simulink model "raspberrypi_I2C_temp_init"  (R2018b)
settings: Solver=FixedStepAuto  StartTime=0.0  StopTime=inf  RelTol=1e-3
undefined symbols (not defined in the file or in its folder): Green, led0
libraries: raspberrypilib x3, embdlinuxlib x1, realtime_examples_misc x1
settings Model: SimulationMode=external  ExtModeTrigDuration=2  Creator=The MathWorks, Inc.  LastModifiedBy=The MathWorks, Inc.
settings SolverCC: PositivePriorityOrder=on
settings DataIOCC: LimitDataPoints=on
settings OptimizationCC: BlockReduction=off  LifeSpan=Inf  MaxStackSize=64
settings DebuggingCC: AllowSymbolicDim=off  SFUnexpectedBacktrackingDiag=warning  SFNoUnconditionalDefaultTransitionDiag=warning  SFExecutionAtInitializationDiag=none
settings HardwareCC: ProdBitPerPointer=32  ProdBitPerSizeT=32  ProdBitPerPtrDiffT=32  ProdLargestAtomicInteger=Long  ProdLargestAtomicFloat=Double  ProdWordSize=32  ProdHWDeviceType=ARM Compatible->ARM Cortex  UseEmbeddedCoderFeatures=off  UseSimulinkCoderFeatures=off
settings ModelReferenceCC: PropagateSignalLabelsOutOfModel=off
settings SFSimCC: SimUseLocalCustomCode=off
settings RTWCC: SystemTargetFile=ert.tlc  HardwareBoard=Raspberry Pi  TemplateMakefile=ert_default_tmf  RTWUseLocalCustomCode=off  Toolchain=GNU GCC Raspberry Pi  BuildConfiguration=Faster Runs
settings CodeAppCC: StateflowObjectComments=on
settings ERTTargetCC: MultiwordLength=2048  ERTCustomFileBanners=off  SupportContinuousTime=on  SupportNonInlinedSFcns=on  RemoveResetFunc=off  SupportVariableSizeSignals=on  ModelStepFunctionPrototypeControlCompliant=off  ConvertIfToSwitch=off  SuppressUnreachableDefaultCases=off
settings ConfigComp: CovMetricSettings=dw  CovHtmlReporting=on  CovSaveCumulativeToWorkspaceVar=on  CovSaveSingleToWorkspaceVar=on  CovExternalEMLEnable=off

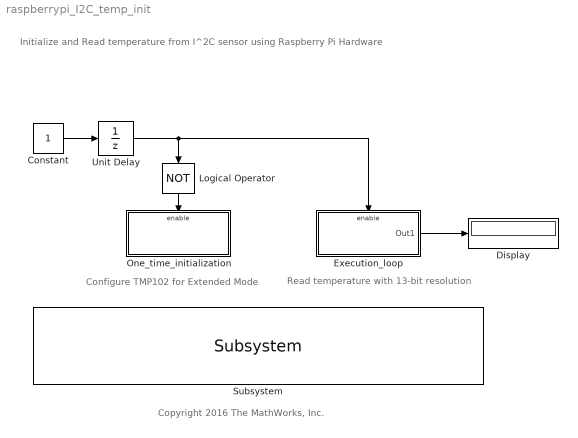
== system raspberrypi_I2C_temp_init ==
  note: Read temperature with 13-bit resolution
  note: Configure TMP102 for Extended Mode
  note: Copyright 2016 The MathWorks, Inc.
  note: Initialize and Read temperature from I^2C sensor
      |  using Raspberry Pi Hardware
  Constant : Constant  OutDataTypeStr=boolean  SampleTime=0.1
  Display : Display
  Execution_loop : Subsystem  TreatAsAtomicUnit=on
  Logical Operator : Logic  Operator=NOT  AllPortsSameDT=off  OutDataTypeStr=boolean
  One_time_initialization : Subsystem  TreatAsAtomicUnit=on
  Subsystem : realtime_examples_misc/Subsystem  SystemSampleTime=-1
  Unit Delay : UnitDelay  SampleTime=-1
  wires:
  Constant/1 -> Unit Delay/1
  Unit Delay/1 -> Execution_loop/Enable, Logical Operator/1
  Logical Operator/1 -> One_time_initialization/Enable
  Execution_loop/1(Out1) -> Display/1

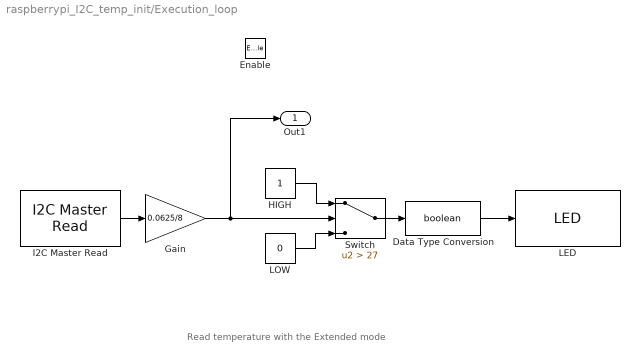
== system raspberrypi_I2C_temp_init/Execution_loop ==
  note: Read temperature with the Extended mode
  Enable : EnablePort
  Data Type Conversion : DataTypeConversion  OutDataTypeStr=boolean
  Gain : Gain  Gain=0.0625/8  OutDataTypeStr=single
  HIGH : Constant  OutDataTypeStr=uint8
  I2C Master Read : raspberrypilib/I2C Master Read  BoardProperty=Pi 3 Model B  Mode=Master  SlaveAddress=hex2dec('48')  SlaveByteOrder=BigEndian  Direction=Receiver  RegisterAddressMode=on  RegisterAddress=0  SlaveDataType=int16  DataLength=1  NoAck=off  RepeatedStart=off  OutputStatus=off  SampleTime=0.1
      settings: SourceProductName=Simulink Support Package for Raspberry Pi Hardware  SourceProductBaseCode=RASPPI
  LED : embdlinuxlib/LED  board=Model B+  led=led0 (Green)  blockPlatform=Raspberry Pi
      settings: SourceProductName=Simulink Support Package for Raspberry Pi Hardware  SourceProductBaseCode=RASPPI
  LOW : Constant  Value=0  OutDataTypeStr=uint8
  Switch : Switch  Criteria=u2 > Threshold  Threshold=27
  Out1 : Outport  InitialOutput=0
  wires:
  LOW/1 -> Switch/3
  Data Type Conversion/1 -> LED/1
  I2C Master Read/1 -> Gain/1
  Gain/1 -> Out1/1, Switch/2
  HIGH/1 -> Switch/1
  Switch/1 -> Data Type Conversion/1

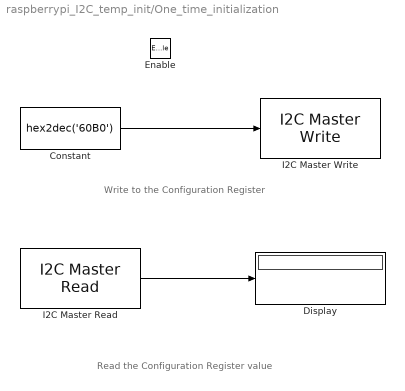
== system raspberrypi_I2C_temp_init/One_time_initialization ==
  note: Write to the Configuration Register
  note: Read the Configuration Register value
  Enable : EnablePort
  Constant : Constant  Value=hex2dec('60B0')  OutDataTypeStr=uint16
  Display : Display
      settings: Format=hex (Stored Integer)
  I2C Master Read : raspberrypilib/I2C Master Read  Priority=2  BoardProperty=Pi 3 Model B  Mode=Master  SlaveAddress=hex2dec( '48' )  SlaveByteOrder=BigEndian  Direction=Receiver  RegisterAddressMode=on  RegisterAddress=1  SlaveDataType=uint16  DataLength=1  NoAck=off  RepeatedStart=off  OutputStatus=off  SampleTime=0.1
      settings: AttributesFormatString=Priority=%<Priority>  SourceProductName=Simulink Support Package for Raspberry Pi Hardware  SourceProductBaseCode=RASPPI
  I2C Master Write : raspberrypilib/I2C Master Write  Priority=1  BoardProperty=Pi 3 Model B  Mode=Master  SlaveAddress=hex2dec('48')  SlaveByteOrder=BigEndian  Direction=Transmitter  RegisterAddressMode=on  RegisterAddress=1  SlaveDataType=uint8  DataLength=1  NoAck=off  RepeatedStart=off  OutputStatus=off
      settings: AttributesFormatString=Priority=%<Priority>  SourceProductName=Simulink Support Package for Raspberry Pi Hardware  SourceProductBaseCode=RASPPI
  wires:
  Constant/1 -> I2C Master Write/1
  I2C Master Read/1 -> Display/1
